simulink model "example_use_sfunctions"  (R2017a)
settings: Solver=FixedStepAuto  StartTime=0.0  StopTime=120  FixedStep=0.01  RelTol=1e-3
libraries: aerolibanimutils x1, dspnetwork x1
settings Model: Creator=Admin  LastModifiedBy=Admin

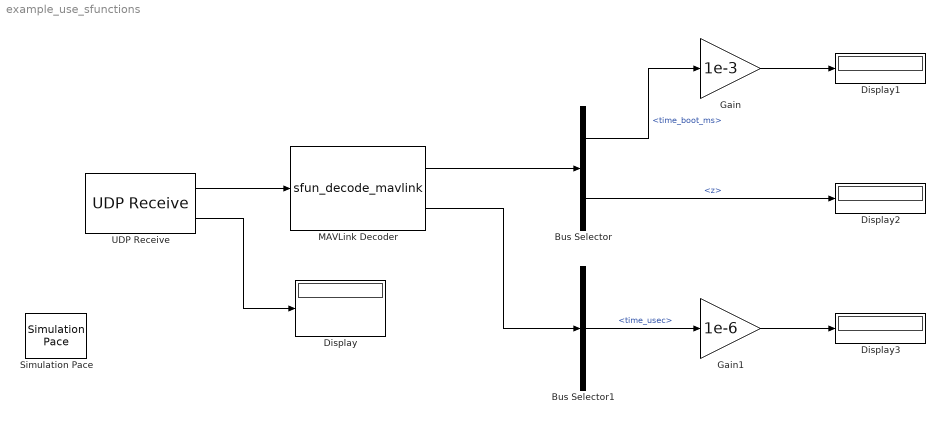
== system example_use_sfunctions ==
  Bus Selector : BusSelector  OutputSignals=time_boot_ms,z
  Bus Selector1 : BusSelector  OutputSignals=time_usec
  Display{,1..3} (4 alike) : Display
  Gain : Gain  Gain=1e-3
  Gain1 : Gain  Gain=1e-6
  MAVLink Decoder : S-Function  FunctionName=sfun_decode_mavlink  SFunctionDeploymentMode=off  EnableBusSupport=off
  Simulation Pace : aerolibanimutils/Simulation Pace  SimulationPace=1  SleepMode=MATLAB Thread  OutputPaceError=off  SampleTime=0.01
  UDP Receive : dspnetwork/UDP Receive  localURL='0.0.0.0'  localPort=25000  remoteURL='0.0.0.0'  remotePort=-1  recvBufferSize=8192  dims=263  signalDatatype=uint8  isVarSize=off  showBlockingTime=on  blockingTime=0  sampletime=0.01  blockPlatform=HOST
  wires:
  UDP Receive/1 -> MAVLink Decoder/1
  UDP Receive/2 -> Display/1
  MAVLink Decoder/1 -> Bus Selector/1
  Bus Selector/1 -> Gain/1  "<time_boot_ms>"
  Bus Selector/2 -> Display2/1  "<z>"
  Gain/1 -> Display1/1
  MAVLink Decoder/2 -> Bus Selector1/1
  Gain1/1 -> Display3/1
  Bus Selector1/1 -> Gain1/1  "<time_usec>"
